simulink model "lin_flexible_steady"  (R2018b)
settings: Solver=ode4  StartTime=0.0  StopTime=10  FixedStep=1/900  RelTol=1e-2  AbsTol=1e-2
undefined symbols (not defined in the file): aircraft, aircraft_visualization, body, fuselage_1_state, ic, wing_1_state, wing_2_state, wing_3_state
libraries: vlm_wing x5, flight_dynamics_models x3, InputBlocks_library x3, OutputBlocks_library x3, aeroelasticity_lib x2, se2a_environment_lib x1, se2a_command_lib x1, flightgear_visualization_lib x1, aerolibfltsims x1, qt_opengl_visualization_lib x1
settings Model: EnablePacing=on  Creator=Yannic  LastModifiedBy=yannic
settings DataIOCC: ExternalInput=[0,trimPoint.Input']  InitialState=trimPoint.State  SaveFormat=Array
settings DebuggingCC: InitInArrayFormatMsg=none

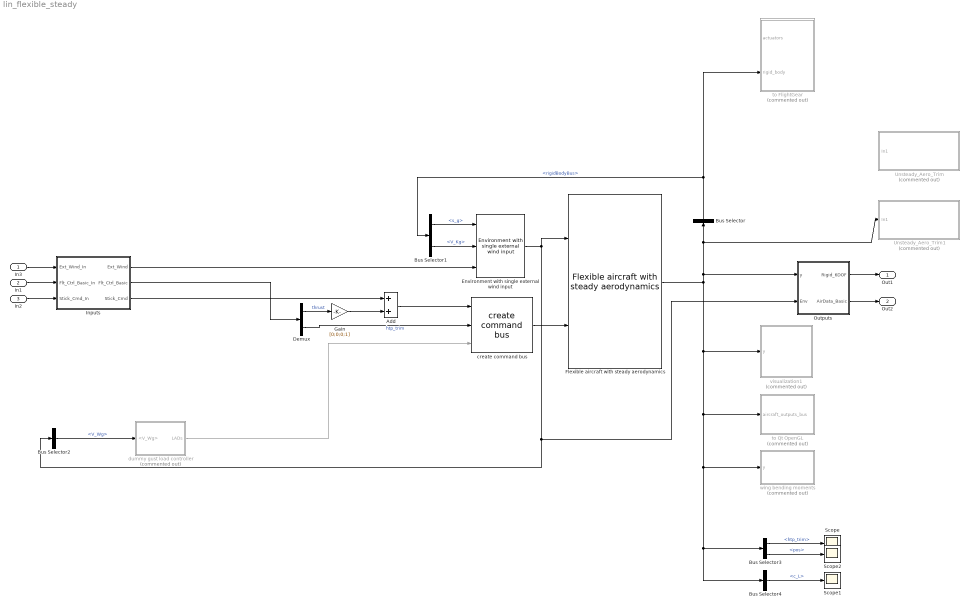
== system lin_flexible_steady ==
  In3 : Inport
  In1 : Inport  Port=2
  In2 : Inport  Port=3
  Add : Sum
  Bus Selector : BusSelector  OutputSignals=flexible_body_bus.rigidBodyBus
  Bus Selector1 : BusSelector  OutputSignals=s_g,V_Kg
  Bus Selector2 : BusSelector  OutputSignals=envir.wind.V_Wg
  Bus Selector3 : BusSelector  OutputSignals=actuators_bus.htp_trim,aeroBus.htp.actuators.pos
  Bus Selector4 : BusSelector  OutputSignals=aeroBus.htp.aero.circulation.c_L
  Demux : Demux  Outputs=2
  Environment with single external wind input : se2a_environment_lib/Environment with single external wind input  aircraft=aircraft  V_A=norm(ic.V_Kb,2)  pos_ref=pos_ref  k_max=1
      settings: SourceProductName=SE2A library
  Flexible aircraft with steady aerodynamics : flight_dynamics_models/Flexible aircraft with steady aerodynamics  aircraft=aircraft  ic=ic
  Gain : Gain  Gain=[0;0;0;1]
  Inputs : Subsystem
  Outputs : Subsystem
  Scope : Scope
  Scope1 : Scope
  Scope2 : Scope
  Unsteady_Aero_Trim : Subsystem  Commented=on
  Unsteady_Aero_Trim1 : Subsystem  Commented=on
  create command bus : se2a_command_lib/create command bus  num_ailerons=aircraft.wing_main.params.num_flaps/2
      settings: SourceProductName=SE2A library
  dummy gust load controller : Subsystem  Commented=on
  to FlightGear : Subsystem  Commented=on
  to Qt OpenGL : Subsystem  Commented=on
  visualization1 : Subsystem  Commented=on
  wing bending moments : Subsystem  Commented=on
  Out1 : Outport
  Out2 : Outport  Port=2
  wires:
  Bus Selector1/1 -> Environment with single external wind input/1  "<s_g>"
  Bus Selector/1 -> to FlightGear/2(rigid_body), Bus Selector1/1  "<rigidBodyBus>"
  Bus Selector2/1 -> dummy gust load controller/1(<V_Wg>)  "<V_Wg>"
  Outputs/1(Rigid_6DOF) -> Out1/1
  Flexible aircraft with steady aerodynamics/1 -> visualization1/1(y), to Qt OpenGL/1(aircraft_outputs_bus), Bus Selector4/1, Bus Selector3/1, wing bending moments/1(y), Unsteady_Aero_Trim1/1(In1), Bus Selector/1, Outputs/1(y)
  Environment with single external wind input/1 -> Outputs/2(Env), Bus Selector2/1, Flexible aircraft with steady aerodynamics/1
  Outputs/2(AirData_Basic) -> Out2/1
  Inputs/1(Ext_Wind) -> Environment with single external wind input/3
  In2/1 -> Inputs/3(Stick_Cmd_In)
  In3/1 -> Inputs/1(Ext_Wind_In)
  dummy gust load controller/1(LADs) -> create command bus/3
  Demux/1 -> Gain/1  "thrust"
  Inputs/3(Stick_Cmd) -> Add/1
  Add/1 -> create command bus/1
  Inputs/2(Flt_Ctrl_Basic) -> Demux/1
  Gain/1 -> Add/2
  Demux/2 -> create command bus/2  "htp_trim"
  create command bus/1 -> Flexible aircraft with steady aerodynamics/2
  Bus Selector1/2 -> Environment with single external wind input/2  "<V_Kg>"
  Bus Selector3/1 -> Scope/1  "<htp_trim>"
  Bus Selector4/1 -> Scope1/1  "<c_L>"
  Bus Selector3/2 -> Scope2/1  "<pos>"
  In1/1 -> Inputs/2(Flt_Ctrl_Basic_In)

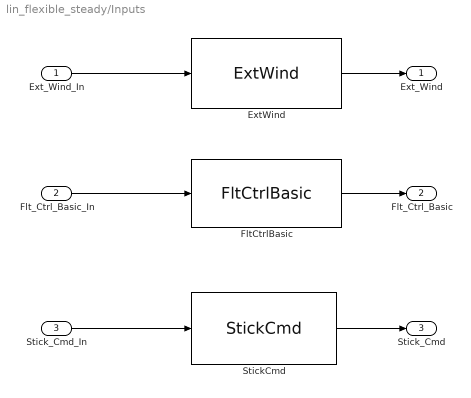
== system lin_flexible_steady/Inputs ==
  Ext_Wind_In : Inport
  Flt_Ctrl_Basic_In : Inport  Port=2
  Stick_Cmd_In : Inport  Port=3
  ExtWind : InputBlocks_library/ExtWind  SystemSampleTime=-1
  FltCtrlBasic : InputBlocks_library/FltCtrlBasic  SystemSampleTime=-1
  StickCmd : InputBlocks_library/StickCmd  SystemSampleTime=-1
  Ext_Wind : Outport
  Flt_Ctrl_Basic : Outport  Port=2
  Stick_Cmd : Outport  Port=3
  wires:
  StickCmd/1 -> Stick_Cmd/1
  FltCtrlBasic/1 -> Flt_Ctrl_Basic/1
  Flt_Ctrl_Basic_In/1 -> FltCtrlBasic/1
  Stick_Cmd_In/1 -> StickCmd/1
  Ext_Wind_In/1 -> ExtWind/1
  ExtWind/1 -> Ext_Wind/1

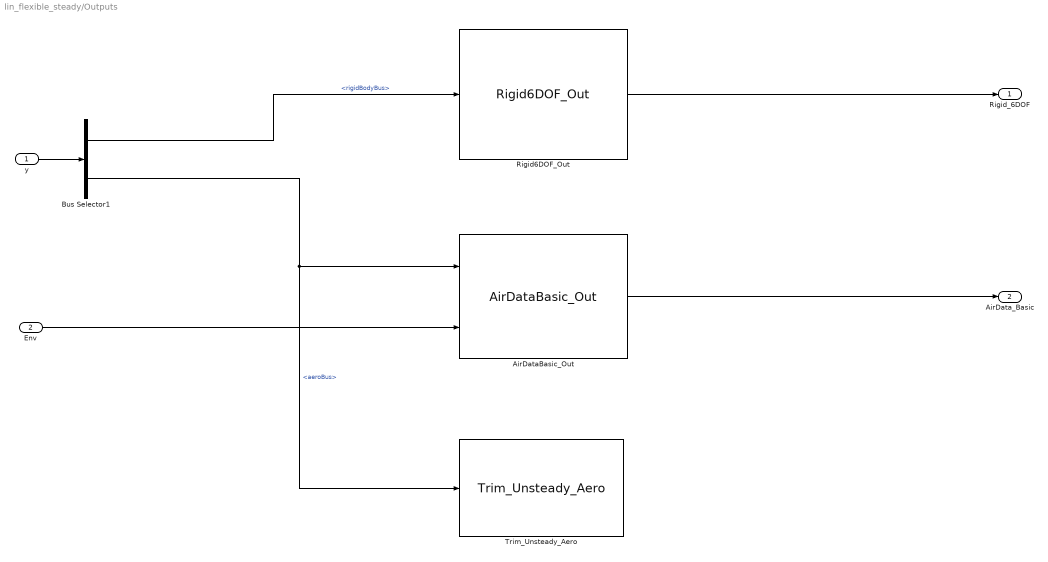
== system lin_flexible_steady/Outputs ==
  y : Inport
  Env : Inport  Port=2
  AirDataBasic_Out : OutputBlocks_library/AirDataBasic_Out
  Bus Selector1 : BusSelector  OutputSignals=flexible_body_bus.rigidBodyBus,aeroBus
  Rigid6DOF_Out : OutputBlocks_library/Rigid6DOF_Out  SystemSampleTime=-1
  Trim_Unsteady_Aero : OutputBlocks_library/Trim_Unsteady_Aero  aircraft=aircraft
  Rigid_6DOF : Outport
  AirData_Basic : Outport  Port=2
  wires:
  y/1 -> Bus Selector1/1
  Bus Selector1/1 -> Rigid6DOF_Out/1  "<rigidBodyBus>"
  Rigid6DOF_Out/1 -> Rigid_6DOF/1
  Env/1 -> AirDataBasic_Out/2
  Bus Selector1/2 -> Trim_Unsteady_Aero/1, AirDataBasic_Out/1  "<aeroBus>"
  AirDataBasic_Out/1 -> AirData_Basic/1

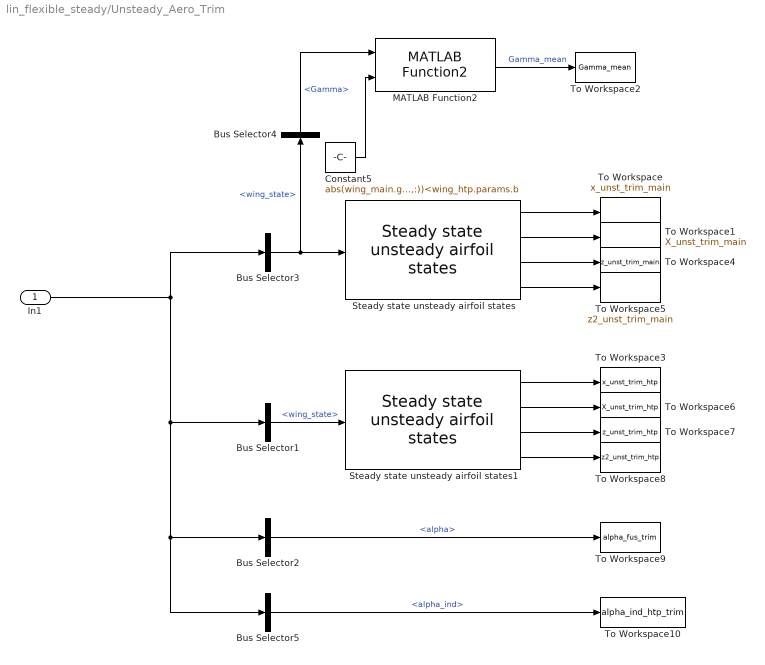
== system lin_flexible_steady/Unsteady_Aero_Trim ==
  In1 : Inport
  Bus Selector1 : BusSelector  OutputSignals=aeroBus.htp.wing_state
  Bus Selector2 : BusSelector  OutputSignals=aeroBus.fuselage.aero.unsteady.alpha
  Bus Selector3 : BusSelector  OutputSignals=aeroBus.main.wing_state
  Bus Selector4 : BusSelector  OutputSignals=aero.circulation.Gamma
  Bus Selector5 : BusSelector  OutputSignals=aeroBus.htp.wing_state.aero.circulation.alpha_ind
  Constant5 : Constant  Value=abs(wing_main.geometry.ctrl_pt.pos(2,:))<wing_htp.params.b
  MATLAB Function2 : flight_dynamics_models/Flexible aircraft with steady aerodynamics/Aerodynamics/MATLAB Function2  SystemSampleTime=-1
      settings: SourceProductName=SE2A library
  Steady state unsteady airfoil states : vlm_wing/Steady state unsteady airfoil states  wing_airfoil=wing_main.airfoil  wing_config=wing_main.config
  Steady state unsteady airfoil states1 : vlm_wing/Steady state unsteady airfoil states  wing_airfoil=wing_htp.airfoil  wing_config=wing_htp.config
  To Workspace : ToWorkspace  VariableName=x_unst_trim_main  SampleTime=-1
      settings: MaxDataPoints=8  Save2DSignal=2-D array (concatenate along first dimension)
  To Workspace1 : ToWorkspace  VariableName=X_unst_trim_main  SampleTime=-1
      settings: MaxDataPoints=3  Save2DSignal=2-D array (concatenate along first dimension)
  To Workspace10 : ToWorkspace  VariableName=alpha_ind_htp_trim  SampleTime=-1
      settings: MaxDataPoints=1  Save2DSignal=2-D array (concatenate along first dimension)
  To Workspace2 : ToWorkspace  VariableName=Gamma_mean  SampleTime=-1
      settings: MaxDataPoints=1
  To Workspace3 : ToWorkspace  VariableName=x_unst_trim_htp  SampleTime=-1
      settings: MaxDataPoints=8  Save2DSignal=2-D array (concatenate along first dimension)
  To Workspace4 : ToWorkspace  VariableName=z_unst_trim_main  SampleTime=-1
      settings: MaxDataPoints=2  Save2DSignal=2-D array (concatenate along first dimension)
  To Workspace5 : ToWorkspace  VariableName=z2_unst_trim_main  SampleTime=-1
      settings: MaxDataPoints=1
  To Workspace6 : ToWorkspace  VariableName=X_unst_trim_htp  SampleTime=-1
      settings: MaxDataPoints=3  Save2DSignal=2-D array (concatenate along first dimension)
  To Workspace7 : ToWorkspace  VariableName=z_unst_trim_htp  SampleTime=-1
      settings: MaxDataPoints=2  Save2DSignal=2-D array (concatenate along first dimension)
  To Workspace8 : ToWorkspace  VariableName=z2_unst_trim_htp  SampleTime=-1
      settings: MaxDataPoints=1
  To Workspace9 : ToWorkspace  VariableName=alpha_fus_trim  SampleTime=-1
      settings: MaxDataPoints=1  Save2DSignal=2-D array (concatenate along first dimension)
  wires:
  Constant5/1 -> MATLAB Function2/2
  Steady state unsteady airfoil states/3 -> To Workspace4/1
  Steady state unsteady airfoil states/2 -> To Workspace1/1
  Bus Selector3/1 -> Steady state unsteady airfoil states/1, Bus Selector4/1  "<wing_state>"
  Bus Selector4/1 -> MATLAB Function2/1  "<Gamma>"
  Steady state unsteady airfoil states/1 -> To Workspace/1
  MATLAB Function2/1 -> To Workspace2/1  "Gamma_mean"
  Steady state unsteady airfoil states/4 -> To Workspace5/1
  Steady state unsteady airfoil states1/4 -> To Workspace8/1
  Steady state unsteady airfoil states1/1 -> To Workspace3/1
  Steady state unsteady airfoil states1/2 -> To Workspace6/1
  Steady state unsteady airfoil states1/3 -> To Workspace7/1
  Bus Selector1/1 -> Steady state unsteady airfoil states1/1  "<wing_state>"
  Bus Selector2/1 -> To Workspace9/1  "<alpha>"
  In1/1 -> Bus Selector5/1, Bus Selector2/1, Bus Selector1/1, Bus Selector3/1
  Bus Selector5/1 -> To Workspace10/1  "<alpha_ind>"

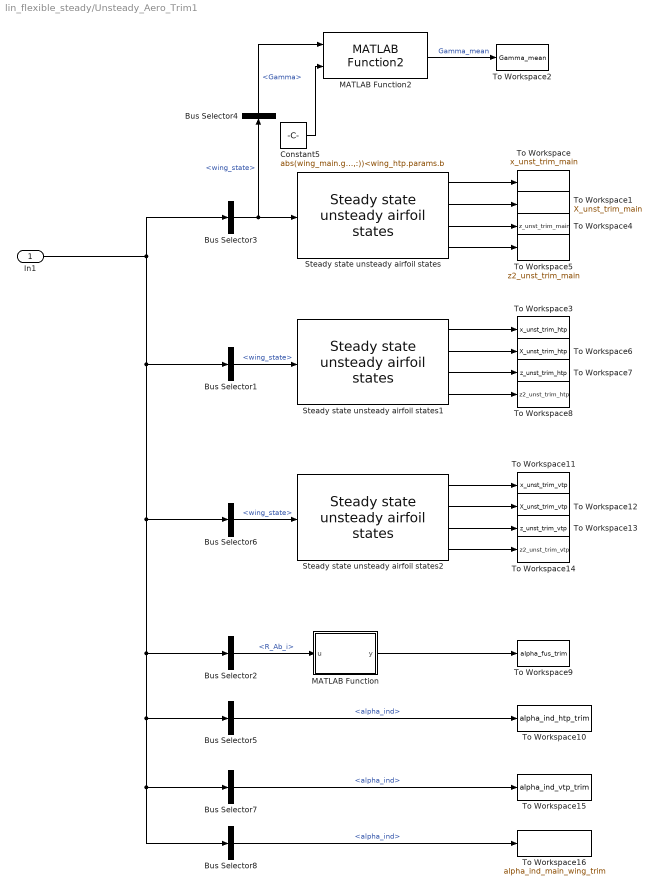
== system lin_flexible_steady/Unsteady_Aero_Trim1 ==
  In1 : Inport
  Bus Selector1 : BusSelector  OutputSignals=aeroBus.htp.wing_state
  Bus Selector2 : BusSelector  OutputSignals=aeroBus.fuselage.aero.R_Ab_i
  Bus Selector3 : BusSelector  OutputSignals=aeroBus.main.wing_state
  Bus Selector4 : BusSelector  OutputSignals=aero.circulation.Gamma
  Bus Selector5 : BusSelector  OutputSignals=aeroBus.htp.wing_state.aero.circulation.alpha_ind
  Bus Selector6 : BusSelector  OutputSignals=aeroBus.vtp.wing_state
  Bus Selector7 : BusSelector  OutputSignals=aeroBus.vtp.wing_state.aero.circulation.alpha_ind
  Bus Selector8 : BusSelector  OutputSignals=aeroBus.main.wing_state.aero.circulation.alpha_ind
  Constant5 : Constant  Value=abs(wing_main.geometry.ctrl_pt.pos(2,:))<wing_htp.params.b
  MATLAB Function : MATLAB Function  TreatAsAtomicUnit=on
  MATLAB Function2 : flight_dynamics_models/Flexible aircraft with steady aerodynamics/Aerodynamics/MATLAB Function2  SystemSampleTime=-1
      settings: SourceProductName=SE2A library
  Steady state unsteady airfoil states : vlm_wing/Steady state unsteady airfoil states  wing_airfoil=wing_main.airfoil  wing_config=wing_main.config
  Steady state unsteady airfoil states1 : vlm_wing/Steady state unsteady airfoil states  wing_airfoil=wing_htp.airfoil  wing_config=wing_htp.config
  Steady state unsteady airfoil states2 : vlm_wing/Steady state unsteady airfoil states  wing_airfoil=wing_vtp.airfoil  wing_config=wing_vtp.config
  To Workspace : ToWorkspace  VariableName=x_unst_trim_main  SampleTime=-1
      settings: MaxDataPoints=8  Save2DSignal=2-D array (concatenate along first dimension)
  To Workspace1 : ToWorkspace  VariableName=X_unst_trim_main  SampleTime=-1
      settings: MaxDataPoints=3  Save2DSignal=2-D array (concatenate along first dimension)
  To Workspace10 : ToWorkspace  VariableName=alpha_ind_htp_trim  SampleTime=-1
      settings: MaxDataPoints=1  Save2DSignal=2-D array (concatenate along first dimension)
  To Workspace11 : ToWorkspace  VariableName=x_unst_trim_vtp  SampleTime=-1
      settings: MaxDataPoints=8  Save2DSignal=2-D array (concatenate along first dimension)
  To Workspace12 : ToWorkspace  VariableName=X_unst_trim_vtp  SampleTime=-1
      settings: MaxDataPoints=3  Save2DSignal=2-D array (concatenate along first dimension)
  To Workspace13 : ToWorkspace  VariableName=z_unst_trim_vtp  SampleTime=-1
      settings: MaxDataPoints=2  Save2DSignal=2-D array (concatenate along first dimension)
  To Workspace14 : ToWorkspace  VariableName=z2_unst_trim_vtp  SampleTime=-1
      settings: MaxDataPoints=1
  To Workspace15 : ToWorkspace  VariableName=alpha_ind_vtp_trim  SampleTime=-1
      settings: MaxDataPoints=1  Save2DSignal=2-D array (concatenate along first dimension)
  To Workspace16 : ToWorkspace  VariableName=alpha_ind_main_wing_trim  SampleTime=-1
      settings: MaxDataPoints=1  Save2DSignal=2-D array (concatenate along first dimension)
  To Workspace2 : ToWorkspace  VariableName=Gamma_mean  SampleTime=-1
      settings: MaxDataPoints=1
  To Workspace3 : ToWorkspace  VariableName=x_unst_trim_htp  SampleTime=-1
      settings: MaxDataPoints=8  Save2DSignal=2-D array (concatenate along first dimension)
  To Workspace4 : ToWorkspace  VariableName=z_unst_trim_main  SampleTime=-1
      settings: MaxDataPoints=2  Save2DSignal=2-D array (concatenate along first dimension)
  To Workspace5 : ToWorkspace  VariableName=z2_unst_trim_main  SampleTime=-1
      settings: MaxDataPoints=1
  To Workspace6 : ToWorkspace  VariableName=X_unst_trim_htp  SampleTime=-1
      settings: MaxDataPoints=3  Save2DSignal=2-D array (concatenate along first dimension)
  To Workspace7 : ToWorkspace  VariableName=z_unst_trim_htp  SampleTime=-1
      settings: MaxDataPoints=2  Save2DSignal=2-D array (concatenate along first dimension)
  To Workspace8 : ToWorkspace  VariableName=z2_unst_trim_htp  SampleTime=-1
      settings: MaxDataPoints=1
  To Workspace9 : ToWorkspace  VariableName=alpha_fus_trim  SampleTime=-1
      settings: MaxDataPoints=1  Save2DSignal=2-D array (concatenate along first dimension)
  wires:
  Constant5/1 -> MATLAB Function2/2
  Steady state unsteady airfoil states/3 -> To Workspace4/1
  Steady state unsteady airfoil states/2 -> To Workspace1/1
  Bus Selector3/1 -> Steady state unsteady airfoil states/1, Bus Selector4/1  "<wing_state>"
  Bus Selector4/1 -> MATLAB Function2/1  "<Gamma>"
  Steady state unsteady airfoil states/1 -> To Workspace/1
  MATLAB Function2/1 -> To Workspace2/1  "Gamma_mean"
  Steady state unsteady airfoil states/4 -> To Workspace5/1
  Steady state unsteady airfoil states1/4 -> To Workspace8/1
  Steady state unsteady airfoil states1/1 -> To Workspace3/1
  Steady state unsteady airfoil states1/2 -> To Workspace6/1
  Steady state unsteady airfoil states1/3 -> To Workspace7/1
  Bus Selector1/1 -> Steady state unsteady airfoil states1/1  "<wing_state>"
  Bus Selector2/1 -> MATLAB Function/1(u)  "<R_Ab_i>"
  Bus Selector5/1 -> To Workspace10/1  "<alpha_ind>"
  In1/1 -> Bus Selector6/1, Bus Selector8/1, Bus Selector7/1, Bus Selector5/1, Bus Selector2/1, Bus Selector1/1, Bus Selector3/1
  Bus Selector6/1 -> Steady state unsteady airfoil states2/1  "<wing_state>"
  Steady state unsteady airfoil states2/3 -> To Workspace13/1
  Steady state unsteady airfoil states2/2 -> To Workspace12/1
  Steady state unsteady airfoil states2/1 -> To Workspace11/1
  Steady state unsteady airfoil states2/4 -> To Workspace14/1
  Bus Selector7/1 -> To Workspace15/1  "<alpha_ind>"
  MATLAB Function/1(y) -> To Workspace9/1
  Bus Selector8/1 -> To Workspace16/1  "<alpha_ind>"

== system lin_flexible_steady/dummy gust load controller ==
  <V_Wg> : Inport
  Gain : Gain  Gain=-0.1*0*ones(1,14)
  Saturation : Saturate  UpperLimit=2  LowerLimit=0
  Scope : Scope
  Selector : Selector  InputPortWidth=3  IndexOptions=Index vector (dialog)  Indices=3  OutputSizes=1
  LADs : Outport
  wires:
  Selector/1 -> Gain/1
  <V_Wg>/1 -> Selector/1
  Saturation/1 -> Scope/1, LADs/1
  Gain/1 -> Saturation/1

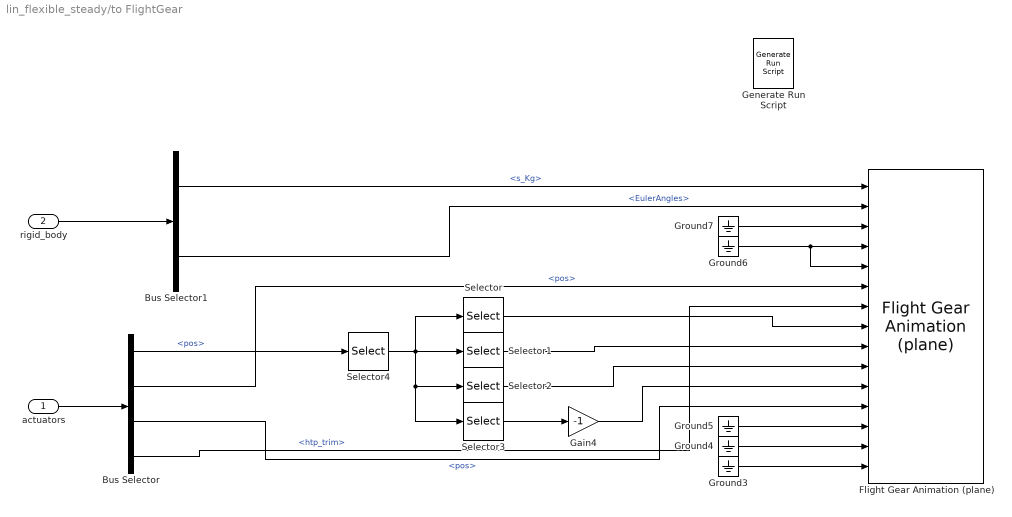
== system lin_flexible_steady/to FlightGear ==
  actuators : Inport
  rigid_body : Inport  Port=2
  Bus Selector : BusSelector  OutputSignals=wings.wing_1.pos,wings.wing_2.pos,wings.wing_3.pos,htp_trim
  Bus Selector1 : BusSelector  OutputSignals=s_Kg,EulerAngles
  Flight Gear Animation (plane) : flightgear_visualization_lib/Flight Gear Animation (plane)  inital_lat=pos_ref.lat  inital_long=pos_ref.lon  inital_height=pos_ref.alt  remoteURL='127.0.0.1'  remotePort=5502
      settings: SourceProductName=LADAC
  Gain4 : Gain  Gain=-1
  Generate Run Script : aerolibfltsims/Generate Run Script  Architecture=Win64  dataFlow=Send  GeometryModelName=777  AirportId=KSFO  RunwayId=10L  InitialAltitude=7224  InitialHeading=113  OffsetDistance=4.72  OffsetAzimuth=0  InstallScenery=off  DisableShaders=off  OriginAddress=127.0.0.1  DestinationPort=5502  OriginPort=5505  LocalAddress=127.0.0.1  OutputFileName=runfg.bat  FlightGearBaseDirectory=C:\Program Files\FlightGear 3.4.0
  Ground{3..7} (5 alike) : Ground
  Selector : Selector  InputPortWidth=6  IndexOptions=Index vector (dialog)  Indices=3  OutputSizes=1
  Selector1 : Selector  InputPortWidth=6  IndexOptions=Index vector (dialog)  Indices=4  OutputSizes=1
  Selector2 : Selector  InputPortWidth=6  IndexOptions=Index vector (dialog)  Indices=1  OutputSizes=1
  Selector3 : Selector  InputPortWidth=6  IndexOptions=Index vector (dialog)  Indices=6  OutputSizes=1
  Selector4 : Selector  InputPortWidth=20  IndexOptions=Index vector (dialog)  Indices=[1:6]  OutputSizes=1
  wires:
  Bus Selector1/2 -> Flight Gear Animation (plane)/2  "<EulerAngles>"
  Bus Selector1/1 -> Flight Gear Animation (plane)/1  "<s_Kg>"
  Bus Selector/3 -> Flight Gear Animation (plane)/12  "<pos>"
  Selector4/1 -> Selector2/1, Selector3/1, Selector/1, Selector1/1
  Selector/1 -> Flight Gear Animation (plane)/8
  Selector1/1 -> Flight Gear Animation (plane)/9
  Selector2/1 -> Flight Gear Animation (plane)/10
  Selector3/1 -> Gain4/1
  Gain4/1 -> Flight Gear Animation (plane)/11
  actuators/1 -> Bus Selector/1
  Bus Selector/1 -> Selector4/1  "<pos>"
  Bus Selector/2 -> Flight Gear Animation (plane)/6  "<pos>"
  Bus Selector/4 -> Flight Gear Animation (plane)/7  "<htp_trim>"
  rigid_body/1 -> Bus Selector1/1
  Ground5/1 -> Flight Gear Animation (plane)/13
  Ground4/1 -> Flight Gear Animation (plane)/14
  Ground3/1 -> Flight Gear Animation (plane)/15
  Ground6/1 -> Flight Gear Animation (plane)/5, Flight Gear Animation (plane)/4
  Ground7/1 -> Flight Gear Animation (plane)/3

== system lin_flexible_steady/to Qt OpenGL ==
  aircraft_outputs_bus : Inport
  Send aircraft bus to Qt OpenGL1 : qt_opengl_visualization_lib/Send aircraft bus to Qt OpenGL  sample_time=1/60  ip_address='localhost'  ip_port=4321  aircraft=aircraft
      settings: SourceProductName=LADAC
  assign aircraft visualization bus : Subsystem  mask{aircraft=aircraft}
      mask prompts: aircraft "aircraft parameters struct"
      mask init:
      | [aircraft_visualization,~,~] ...
      |     = aircraftCreateVisualizer(aircraft);
      | struct2bus(aircraft_visualization,'aircraft_visualization_bus');
      mask DialogControl DescGroupVar Prompt: Assign aircraft visualization bus
  wires:
  aircraft_outputs_bus/1 -> assign aircraft visualization bus/1(aircraft_outputs_bus)
  assign aircraft visualization bus/1(aircraft_visualization_bus) -> Send aircraft bus to Qt OpenGL1/1

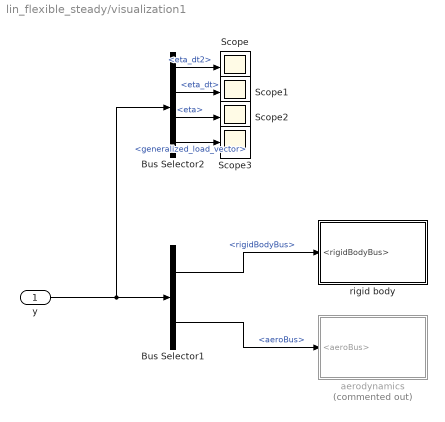
== system lin_flexible_steady/visualization1 ==
  y : Inport
  Bus Selector1 : BusSelector  OutputSignals=flexible_body_bus.rigidBodyBus,aeroBus
  Bus Selector2 : BusSelector  OutputSignals=flexible_body_bus.eta_dt2,flexible_body_bus.eta_dt,flexible_body_bus.eta,flexible_body_bus.generalized_load_vector
  Scope{,1..3} (4 alike) : Scope
  aerodynamics : Subsystem  Commented=on
  rigid body : Subsystem
  wires:
  y/1 -> Bus Selector2/1, Bus Selector1/1
  Bus Selector1/1 -> rigid body/1(<rigidBodyBus>)  "<rigidBodyBus>"
  Bus Selector1/2 -> aerodynamics/1(<aeroBus>)  "<aeroBus>"
  Bus Selector2/4 -> Scope3/1  "<generalized_load_vector>"
  Bus Selector2/3 -> Scope2/1  "<eta>"
  Bus Selector2/2 -> Scope1/1  "<eta_dt>"
  Bus Selector2/1 -> Scope/1  "<eta_dt2>"

== system lin_flexible_steady/wing bending moments ==
  y : Inport
  Bus Selector4 : BusSelector  OutputSignals=structureBus.x,aeroBus.main.R_i_Ab
  Scope : Scope  NumInputPorts=2
  wing dynamic bending moment1 : aeroelasticity_lib/wing dynamic bending moment  structure=structure  structure_red=structure_red  eta=[-0.9:0.2:0.9]
      settings: SourceProductName=LADAC
  wing static bending moment1 : aeroelasticity_lib/wing static bending moment  wing_main=wing_main  structure=structure  eta=[-0.9:0.2:0.9]
      settings: SourceProductName=LADAC
  wires:
  Bus Selector4/1 -> wing dynamic bending moment1/1  "<x>"
  y/1 -> Bus Selector4/1
  wing dynamic bending moment1/1 -> Scope/1
  wing static bending moment1/1 -> Scope/2
  Bus Selector4/2 -> wing static bending moment1/1  "<R_i_Ab>"

== system lin_flexible_steady/to Qt OpenGL/assign aircraft visualization bus ==
  aircraft_outputs_bus : Inport
  Bus Assignment : BusAssignment  AssignedSignals=wing_1_state,wing_2_state,wing_3_state,fuselage_1_state,body
  Bus Selector3 : BusSelector  OutputSignals=aeroBus.main,aeroBus.htp,aeroBus.vtp,aeroBus.fuselage,flexible_body_bus.rigidBodyBus
  Constant1 : Constant  Value=aircraft_visualization  OutDataTypeStr=Bus: aircraft_visualization_bus
  aircraft_visualization_bus : Outport
  wires:
  Bus Assignment/1 -> aircraft_visualization_bus/1
  aircraft_outputs_bus/1 -> Bus Selector3/1
  Constant1/1 -> Bus Assignment/1
  Bus Selector3/1 -> Bus Assignment/2  "<main>"
  Bus Selector3/2 -> Bus Assignment/3  "<htp>"
  Bus Selector3/4 -> Bus Assignment/5  "<fuselage>"
  Bus Selector3/3 -> Bus Assignment/4  "<vtp>"
  Bus Selector3/5 -> Bus Assignment/6  "<rigidBodyBus>"

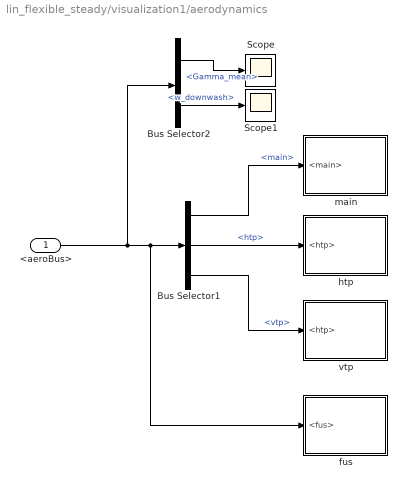
== system lin_flexible_steady/visualization1/aerodynamics ==
  <aeroBus> : Inport
  Bus Selector1 : BusSelector  OutputSignals=main,htp,vtp
  Bus Selector2 : BusSelector  OutputSignals=downwash.Gamma_mean,downwash.w_downwash
  Scope : Scope
  Scope1 : Scope
  fus : Subsystem
  htp : Subsystem
  main : Subsystem
  vtp : Subsystem
  wires:
  <aeroBus>/1 -> Bus Selector2/1, fus/1(<fus>), Bus Selector1/1
  Bus Selector1/2 -> htp/1(<htp>)  "<htp>"
  Bus Selector1/1 -> main/1(<main>)  "<main>"
  Bus Selector1/3 -> vtp/1(<htp>)  "<vtp>"
  Bus Selector2/2 -> Scope1/1  "<w_downwash>"
  Bus Selector2/1 -> Scope/1  "<Gamma_mean>"

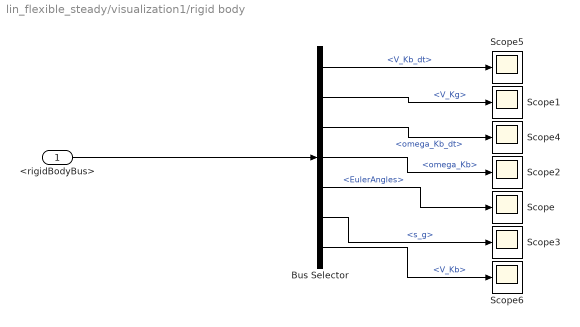
== system lin_flexible_steady/visualization1/rigid body ==
  <rigidBodyBus> : Inport
  Bus Selector : BusSelector  OutputSignals=V_Kb_dt,V_Kg,omega_Kb_dt,omega_Kb,EulerAngles,s_g,V_Kb
  Scope{,1..6} (7 alike) : Scope
  wires:
  Bus Selector/5 -> Scope/1  "<EulerAngles>"
  Bus Selector/2 -> Scope1/1  "<V_Kg>"
  Bus Selector/6 -> Scope3/1  "<s_g>"
  Bus Selector/4 -> Scope2/1  "<omega_Kb>"
  <rigidBodyBus>/1 -> Bus Selector/1
  Bus Selector/3 -> Scope4/1  "<omega_Kb_dt>"
  Bus Selector/1 -> Scope5/1  "<V_Kb_dt>"
  Bus Selector/7 -> Scope6/1  "<V_Kb>"

== system lin_flexible_steady/visualization1/aerodynamics/fus ==
  <fus> : Inport
  Bus Selector : BusSelector  OutputSignals=fuselage.aero.R_Ab,fuselage.aero.Q_Ab,fuselage.aero.unsteady.alpha_dt,fuselage.aero.unsteady.beta_dt,fuselage.aero.unsteady.alpha,fuselage.aero.unsteady.beta
  Scope{,1..5} (6 alike) : Scope
  wires:
  <fus>/1 -> Bus Selector/1
  Bus Selector/4 -> Scope3/1  "<beta_dt>"
  Bus Selector/3 -> Scope2/1  "<alpha_dt>"
  Bus Selector/1 -> Scope1/1  "<R_Ab>"
  Bus Selector/2 -> Scope/1  "<Q_Ab>"
  Bus Selector/6 -> Scope4/1  "<beta>"
  Bus Selector/5 -> Scope5/1  "<alpha>"

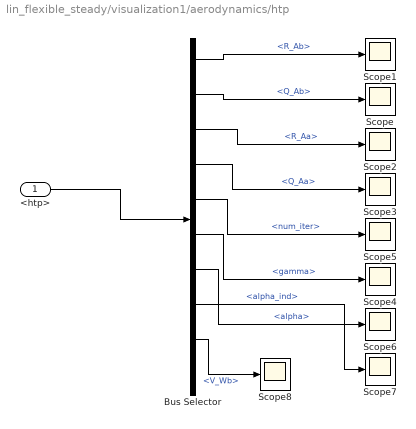
== system lin_flexible_steady/visualization1/aerodynamics/htp ==
  <htp> : Inport
  Bus Selector : BusSelector  OutputSignals=R_Ab,Q_Ab,R_Aa,Q_Aa,num_iter,wing_state.aero.circulation.gamma,wing_state.body.alpha,wing_state.aero.circulation.alpha_ind,wing_state.external.V_Wb,wing_state.aero.coeff_loc.c_XYZ_b
  Scope{,1..8} (9 alike) : Scope
  wires:
  <htp>/1 -> Bus Selector/1
  Bus Selector/4 -> Scope3/1  "<Q_Aa>"
  Bus Selector/3 -> Scope2/1  "<R_Aa>"
  Bus Selector/1 -> Scope1/1  "<R_Ab>"
  Bus Selector/2 -> Scope/1  "<Q_Ab>"
  Bus Selector/6 -> Scope4/1  "<gamma>"
  Bus Selector/5 -> Scope5/1  "<num_iter>"
  Bus Selector/7 -> Scope6/1  "<alpha>"
  Bus Selector/8 -> Scope7/1  "<alpha_ind>"
  Bus Selector/9 -> Scope8/1  "<V_Wb>"

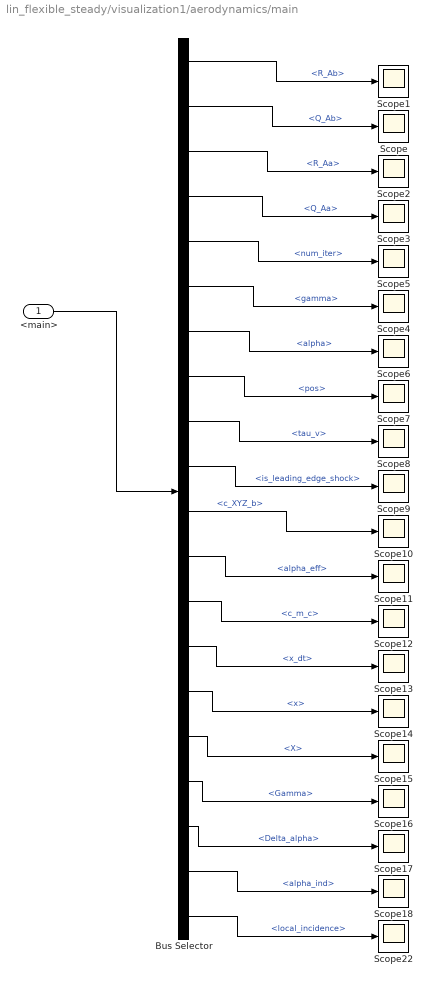
== system lin_flexible_steady/visualization1/aerodynamics/main ==
  <main> : Inport
  Bus Selector : BusSelector  OutputSignals=R_Ab,Q_Ab,R_Aa,Q_Aa,num_iter,wing_state.aero.circulation.gamma,wing_state.body.alpha,wing_state.actuators.pos,wing_state.aero.unsteady.tau_v,wing_state.aero.unsteady.is_leading_edge_shock,wing_state.aero.coeff_loc.c_XYZ_b,wing_state.aero.circulation.alpha_eff,wing_state.aero.unsteady.c_m_c,wing_state.aero.unsteady.x_dt,wing_state.aero.unsteady.x,wing_state.aero.unsteady.X,wing_state.aero.circulation.Gamma,wing_state.aero.circulation.Delta_alpha,wing_state.aero.circulation.alpha_ind,wing_state.geometry.ctrl_pt.local_incidence
  Scope{,1..18,22} (20 alike) : Scope
  wires:
  Bus Selector/5 -> Scope5/1  "<num_iter>"
  Bus Selector/6 -> Scope4/1  "<gamma>"
  Bus Selector/2 -> Scope/1  "<Q_Ab>"
  Bus Selector/1 -> Scope1/1  "<R_Ab>"
  Bus Selector/3 -> Scope2/1  "<R_Aa>"
  Bus Selector/4 -> Scope3/1  "<Q_Aa>"
  <main>/1 -> Bus Selector/1
  Bus Selector/7 -> Scope6/1  "<alpha>"
  Bus Selector/8 -> Scope7/1  "<pos>"
  Bus Selector/9 -> Scope8/1  "<tau_v>"
  Bus Selector/10 -> Scope9/1  "<is_leading_edge_shock>"
  Bus Selector/12 -> Scope11/1  "<alpha_eff>"
  Bus Selector/13 -> Scope12/1  "<c_m_c>"
  Bus Selector/14 -> Scope13/1  "<x_dt>"
  Bus Selector/15 -> Scope14/1  "<x>"
  Bus Selector/16 -> Scope15/1  "<X>"
  Bus Selector/17 -> Scope16/1  "<Gamma>"
  Bus Selector/18 -> Scope17/1  "<Delta_alpha>"
  Bus Selector/19 -> Scope18/1  "<alpha_ind>"
  Bus Selector/11 -> Scope10/1  "<c_XYZ_b>"
  Bus Selector/20 -> Scope22/1  "<local_incidence>"

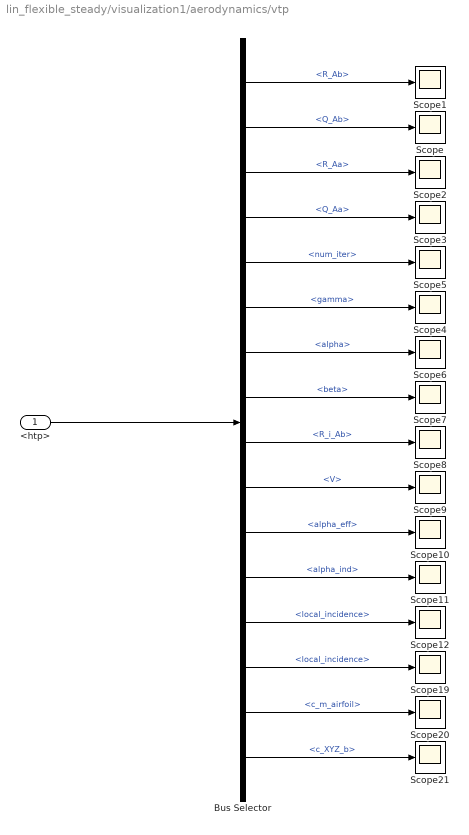
== system lin_flexible_steady/visualization1/aerodynamics/vtp ==
  <htp> : Inport
  Bus Selector : BusSelector  OutputSignals=R_Ab,Q_Ab,R_Aa,Q_Aa,num_iter,wing_state.aero.circulation.gamma,wing_state.body.alpha,wing_state.body.beta,R_i_Ab,wing_state.aero.local_inflow.V,wing_state.aero.circulation.alpha_eff,wing_state.aero.circulation.alpha_ind,wing_state.geometry.ctrl_pt_dt.local_incidence,wing_state.geometry.ctrl_pt.local_incidence,wing_state.aero.coeff_loc.c_m_airfoil,wing_state.aero.coeff_loc.c_XYZ_b
  Scope{,1..12,19..21} (16 alike) : Scope
  wires:
  Bus Selector/5 -> Scope5/1  "<num_iter>"
  Bus Selector/6 -> Scope4/1  "<gamma>"
  Bus Selector/2 -> Scope/1  "<Q_Ab>"
  Bus Selector/1 -> Scope1/1  "<R_Ab>"
  Bus Selector/3 -> Scope2/1  "<R_Aa>"
  Bus Selector/4 -> Scope3/1  "<Q_Aa>"
  <htp>/1 -> Bus Selector/1
  Bus Selector/7 -> Scope6/1  "<alpha>"
  Bus Selector/8 -> Scope7/1  "<beta>"
  Bus Selector/9 -> Scope8/1  "<R_i_Ab>"
  Bus Selector/10 -> Scope9/1  "<V>"
  Bus Selector/11 -> Scope10/1  "<alpha_eff>"
  Bus Selector/12 -> Scope11/1  "<alpha_ind>"
  Bus Selector/14 -> Scope19/1  "<local_incidence>"
  Bus Selector/15 -> Scope20/1  "<c_m_airfoil>"
  Bus Selector/16 -> Scope21/1  "<c_XYZ_b>"
  Bus Selector/13 -> Scope12/1  "<local_incidence>"

== matlab function lin_flexible_steady/Unsteady_Aero_Trim1/MATLAB Function ==
  data: u input; y output
function y = fcn(u)

y = u(3,:);
